simulink model "Active_Cell_BMS"  (R2024a)
settings: Solver=VariableStepAuto  StartTime=0.0  StopTime=10.0  RelTol=1e-3
undefined symbols (not defined in the file): Ion, Lithium
libraries: spsIdealSwitchLib x10, spsDiodeLib x8, spsBatteryLib x4, spsSeriesRLCBranchLib x2, spsDCVoltageSourceLib x1, spsPWMGenerator2LevelLib x1, sps_lib x1
settings Model: Creator=RGUKT  LastModifiedBy=RGUKT

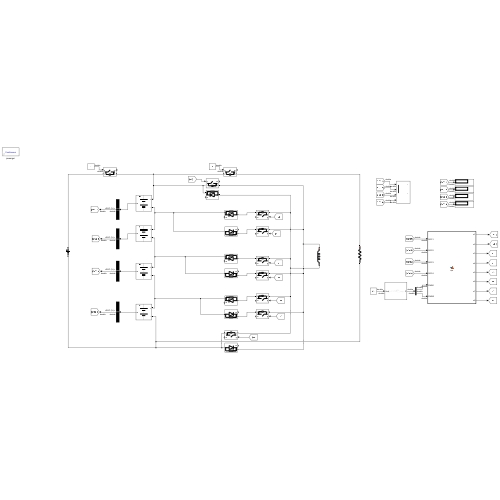
[thumbnail: Simulink's stored preview of the top-level diagram]
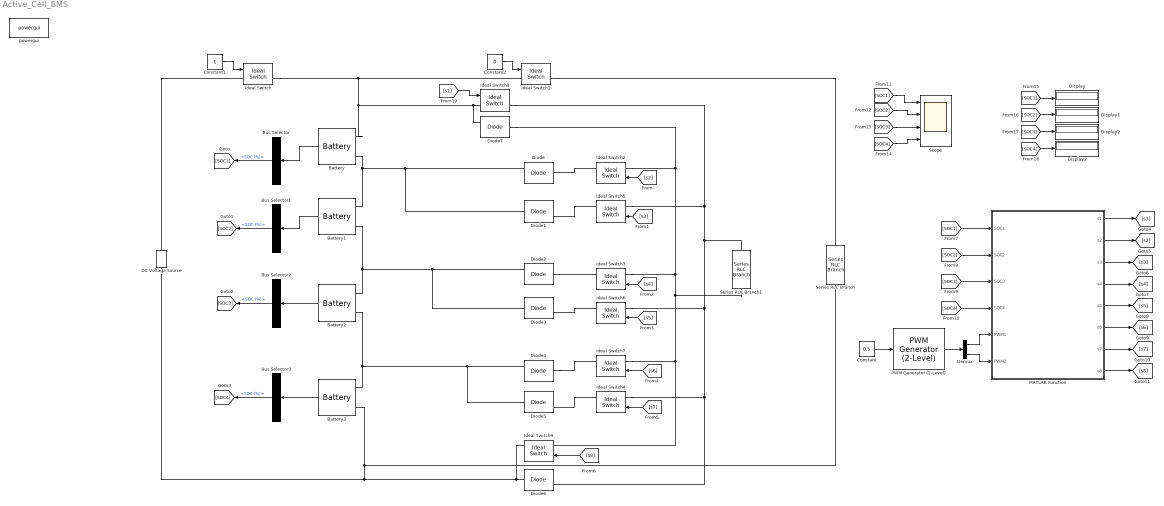
== system Active_Cell_BMS ==
  Battery{,1..3} (4 alike) : spsBatteryLib/Battery  BatType=Lithium-Ion  ShowTempParam=off  ThermalPreset=no  ShowAgeParam=off  NomV=7.2  NomQ=5.4  SOC=100  Batt_Tr=30  PresetModel=on  MaxQ=5.4  MinV=5.4  FullV=8.3807  Dis_rate=2.3478  R=0.013333  Normal_OP=4.8835  expZone="[7.7788      0.2653]"  current=[6.5 13 32.5]  Units=Time  Tci=20  NomT=20  T2=-30  MaxQ2=4.8  FullV2=7.1  Normal_OP2=5.655  expZone2="[6.58           1]"  Rca=0.6  ti=2000  Dp=0  Neq0=0  Tsim=1e6  Ta1=25  Qeol=5.4*0.9  Reol=0.013333*1.2  Char_age=[2.3478, 3]  Dis_age=[2.3478, 10]  N1=1500  N2=10500  N3=1000  N4=1400  Ta2=45  N5=950
  Bus Selector{,1..3} (4 alike) : BusSelector  OutputSignals=SOC (%)
  Constant : Constant  Value=0.5
  Constant1 : Constant
  Constant2 : Constant  Value=0
  DC Voltage Source : spsDCVoltageSourceLib/DC Voltage Source  Amplitude=100  Measurements=None
  Demux : Demux  Outputs=2
  Diode{,1..7} (8 alike) : spsDiodeLib/Diode  Ron=0.001  Lon=0  Vf=0.8  IC=0  UseSnubber=0  Rs=500  Cs=250e-9  Measurements=on
  Display{,1..3} (4 alike) : Display
  Ideal Switch{,1..9} (10 alike) : spsIdealSwitchLib/Ideal Switch  Ron=0.001  Lon=0  IC=0  Rs=1e5  Cs=inf  Measurements=on
  MATLAB Function : MATLAB Function  TreatAsAtomicUnit=on
  PWM Generator (2-Level) : spsPWMGenerator2LevelLib/PWM Generator (2-Level)  ModulatorType=Single-phase full-bridge (4 pulses)  ModulatorMode=Unsynchronized  Fc=27*60  Pc=90  nF=27  MinMax="[ -1  1 ]"  SamplingTechnique=Natural  ModulatingSignals=off  m=0.8  Freq=60  Phase=0  Ts=0  ShowCarrierOutport=off
  Scope : Scope  NumInputPorts=4
  Series RLC Branch : spsSeriesRLCBranchLib/Series RLC Branch  LConnTagsString=__new0  RConnTagsString=__new0  BranchType=R  Resistance=1  Inductance=1e-3  SetiL0=off  InitialCurrent=0  Capacitance=1e-6  Setx0=off  InitialVoltage=0  Measurements=None
  Series RLC Branch1 : spsSeriesRLCBranchLib/Series RLC Branch  LConnTagsString=__new0  RConnTagsString=__new0  BranchType=L  Resistance=1  Inductance=1e-3  SetiL0=off  InitialCurrent=0  Capacitance=1e-6  Setx0=off  InitialVoltage=0  Measurements=None
  powergui : sps_lib/powergui  Priority=1  SimulationMode=Continuous  SampleTime=50e-6  frequency=60  Iterations=50  frequencyindice=0  Pbase=100e6  ErrMax=1e-4  UnitsV=kV  UnitsW=MW  buscounter=0  FunctionMessages=off  echomessages=off  EnableUseOfTLC=off  CurrentSourceSwitches=off  DisableSnubberDevices=off  DisableRonSwitches=off  DisableVfSwitches=off  DisplayEquations=off  AutomaticDiscreteSolvers=off  SolverType=Tustin/Backward Euler (TBE)  Interpol=off  ExternalGateDelay=off  methode=off  Ts=100  x0status=blocks  SPID=on  SwTol=0  HookPort=off  NonlinearTolerance=1e-4  nMaxIteration=100  ContinueOnMaxIteration=off  RestoreLinks=warning  ResistiveCurrentMeasurement=off  Frange=[0:2:500]  Ylog=off  Xlog=on  ShowGrid=off  save=off  variable=ZData  structure=0  ZoomFFT=off  StartTime=0.0  cycles=1  DisplayStyle=1  fundamental=60  FreqAxis=off  MaxFrequency=1000  frequencyindicesteady=1  RmsSteady=1  display=off
  wires:
  Battery/1 -> Bus Selector/1
  Battery1/1 -> Bus Selector1/1
  Battery2/1 -> Bus Selector2/1
  Battery3/1 -> Bus Selector3/1
  Bus Selector/1 -> [SOC1]  "<SOC (%)>"
  Bus Selector3/1 -> [SOC4]  "<SOC (%)>"
  Bus Selector2/1 -> [SOC3]  "<SOC (%)>"
  Bus Selector1/1 -> [SOC2]  "<SOC (%)>"
  [s2] -> Ideal Switch2/1
  [s3] -> Ideal Switch5/1
  [s5] -> Ideal Switch6/1
  [s4] -> Ideal Switch3/1
  [s6] -> Ideal Switch7/1
  [s7] -> Ideal Switch4/1
  [s8] -> Ideal Switch9/1
  [SOC1] -> MATLAB Function/1(SOC1)
  PWM Generator (2-Level)/1 -> Demux/1
  Demux/1 -> MATLAB Function/5(PWM1)
  [SOC2] -> MATLAB Function/2(SOC2)
  [SOC3] -> MATLAB Function/3(SOC3)
  [SOC4] -> MATLAB Function/4(SOC4)
  Demux/2 -> MATLAB Function/6(PWM2)
  [SOC1] -> Scope/1
  [SOC2] -> Scope/2
  [SOC3] -> Scope/3
  [SOC4] -> Scope/4
  [SOC1] -> Display/1
  [SOC2] -> Display1/1
  [SOC3] -> Display2/1
  [SOC4] -> Display3/1
  MATLAB Function/1(s1) -> [s1]
  MATLAB Function/2(s2) -> [s2]
  MATLAB Function/3(s3) -> [s3]
  MATLAB Function/4(s4) -> [s4]
  MATLAB Function/5(s5) -> [s5]
  MATLAB Function/6(s6) -> [s6]
  MATLAB Function/7(s7) -> [s7]
  MATLAB Function/8(s8) -> [s8]
  [s1] -> Ideal Switch8/1
  Constant1/1 -> Ideal Switch/1
  Constant2/1 -> Ideal Switch1/1
  Constant/1 -> PWM Generator (2-Level)/1
  connections:
  Battery/LConn2 -- Diode1/LConn1 -- Diode/RConn1 -- Battery1/LConn1
  Battery1/LConn2 -- Diode3/LConn1 -- Diode2/RConn1 -- Battery2/LConn1
  Battery2/LConn2 -- Diode5/LConn1 -- Diode4/RConn1 -- Battery3/LConn1
  DC Voltage Source/RConn1 -- Ideal Switch/LConn1
  Ideal Switch/RConn1 -- Diode7/RConn1 -- Ideal Switch8/LConn1 -- Battery/LConn1 -- Ideal Switch1/LConn1
  Ideal Switch1/RConn1 -- Series RLC Branch/LConn1
  Ideal Switch2/RConn1 -- Diode/LConn1
  Ideal Switch5/RConn1 -- Diode1/RConn1
  Ideal Switch3/RConn1 -- Diode2/LConn1
  Ideal Switch6/RConn1 -- Diode3/RConn1
  Diode4/LConn1 -- Ideal Switch7/RConn1
  Ideal Switch4/RConn1 -- Diode5/RConn1
  Ideal Switch8/RConn1 -- Ideal Switch5/LConn1 -- Series RLC Branch1/LConn1 -- Ideal Switch4/LConn1 -- Diode6/RConn1 -- Ideal Switch6/LConn1
  DC Voltage Source/LConn1 -- Battery3/LConn2 -- Series RLC Branch/RConn1 -- Ideal Switch9/RConn1 -- Diode6/LConn1
  Diode7/LConn1 -- Ideal Switch2/LConn1 -- Ideal Switch3/LConn1 -- Series RLC Branch1/RConn1 -- Ideal Switch7/LConn1 -- Ideal Switch9/LConn1

== matlab function Active_Cell_BMS/MATLAB Function ==
  data: SOC1 input; s1 output; SOC2 input; SOC3 input; SOC4 input; PWM1 input; PWM2 input; s2 output; s3 output; s4 output; s5 output; s6 output; s7 output; s8 output
function [s1,s2,s3,s4,s5,s6,s7,s8] = fcn(SOC1,SOC2,SOC3,SOC4,PWM1,PWM2)
High = max([SOC1,SOC2,SOC3,SOC4]);
Low =  min([SOC1,SOC2,SOC3,SOC4]);
if High==SOC1&&Low==SOC2
    s1=PWM1;s2=1;s5=PWM2;
    s3=0;s4=0;s6=0;s7=0;s8=0;

elseif High==SOC1&&Low==SOC3
    s1=PWM1;s2=PWM1;s4=PWM2;s7=PWM2;
    s3=0;s5=0;s6=0;s8=0;

elseif High==SOC1&&Low==SOC4
    s1=PWM1;s2=PWM2;s6=PWM2;
    s3=0;s4=0;s5=0;s7=0;s8=0;

elseif High==SOC2&&Low==SOC1
    s3=1;s4=PWM1;
    s1=0;s2=0;s5=0;s6=0;s7=0;s8=0;

elseif High==SOC2&&Low==SOC3
    s3=PWM1;s4=PWM1;s7=PWM2;
    s1=0;s2=0;s5=0;s6=0;s8=0;

elseif High==SOC2&&Low==SOC4
    s3=PWM1;s4=PWM1;s6=PWM2;
    s1=0;s2=0;s5=0;s7=0;s8=0;

elseif High==SOC3&&Low==SOC1
    s3=PWM2;s5=PWM1;s6=PWM1;
    s1=0;s2=0;s4=0;s7=0;s8=0;

elseif High==SOC3&&Low==SOC2
    s2=PWM2;s5=1;s6=PWM1;
    s1=0;s3=0;s4=0;s7=0;s8=0;
elseif High==SOC3&&Low==SOC4
    s5=PWM1;s6=1;
    s1=0;s2=0;s3=0;s4=0;s7=0;s8=0;

elseif High==SOC4&&Low==SOC1
    s3=PWM2;s7=PWM1;s8=PWM1;
    s1=0;s2=0;s4=0;s5=0;s6=0;
elseif High==SOC4&&Low==SOC2
    s2=PWM2;s5=PWM2;s7=PWM1;s8=PWM1;
    s1=0;s3=0;s4=0;s6=0;
elseif High==SOC4&&Low==SOC3
    s4=PWM2;s8=PWM1;s7=1;
    s1=0;s2=0;s3=0;s5=0;s6=0;
    
else
    s1=0;
    s2=0;
    s3=0;
    s4=0;
    s5=0;
    s6=0;
    s7=0;
    s8=0;
end
end
